simulink model "problem2"  (R2016a)
settings: Solver=VariableStepAuto  StartTime=0.0  StopTime=10.0  RelTol=1e-3
values from neighbouring files (symbols this model uses):
  x_path = planTraj(x2_i(1),x2_f(1),time)    [main.m]    (also in main_1.m = planTraj(x2_i(1),x2_f(1), 10); main_3.m = planTraj(x2_i(1),x2_f(1),10); test.m)
  y_path = planTraj(x2_i(2),x2_f(2),time)    [main.m]    (also in main_1.m = planTraj(x2_i(2),x2_f(2),10); main_3.m = planTraj(x2_i(2),x2_f(2),10); test.m)
libraries: dspinverses x1
settings Model: Creator=nathaniel  LastModifiedBy=nathaniel
settings GRTTargetCC: GeneratePreprocessorConditionals=Use local settings

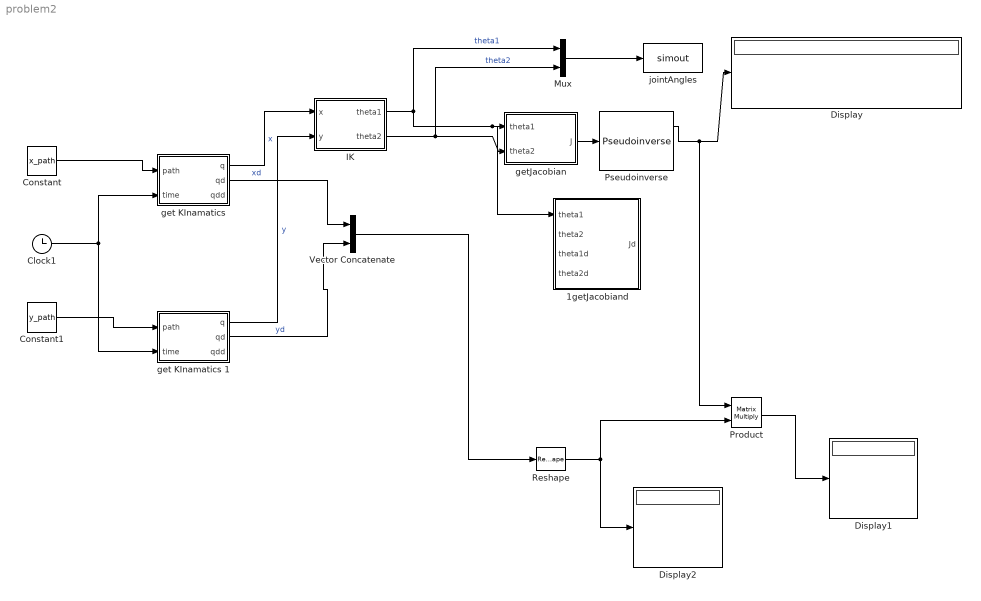
== system problem2 ==
  " 1getJacobiand " : MATLAB Function  TreatAsAtomicUnit=on
  Clock1 : Clock
  Constant : Constant  Value=x_path
  Constant1 : Constant  Value=y_path
  Display : Display
  Display1 : Display
  Display2 : Display
  "IK " : MATLAB Function  TreatAsAtomicUnit=on
  Mux : Mux  Inputs=2
  Product : Product  Multiplication=Matrix(*)
  Pseudoinverse : dspinverses/Pseudoinverse  wanterr=on
  Reshape : Reshape  OutputDimensionality=Column vector (2-D)
  Vector Concatenate : Concatenate
  "get KInamatics " : MATLAB Function  TreatAsAtomicUnit=on
  get KInamatics 1 : MATLAB Function  TreatAsAtomicUnit=on
  getJacobian : MATLAB Function  TreatAsAtomicUnit=on
  jointAngles : ToWorkspace  VariableName=simout  SaveFormat=Structure With Time  SampleTime=-1
  wires:
  Clock1/1 -> get KInamatics 1/2(time), "get KInamatics "/2(time)
  Constant1/1 -> get KInamatics 1/1(path)
  Constant/1 -> "get KInamatics "/1(path)
  get KInamatics 1/1(q) -> "IK "/2(y)  "y"
  "get KInamatics "/1(q) -> "IK "/1(x)  "x"
  "IK "/1(theta1) -> " 1getJacobiand "/1(theta1), getJacobian/1(theta1), Mux/1  "theta1"
  "IK "/2(theta2) -> getJacobian/2(theta2), Mux/2  "theta2"
  getJacobian/1(J) -> Pseudoinverse/1
  Pseudoinverse/1 -> Product/1, Display/1
  Mux/1 -> jointAngles/1
  "get KInamatics "/2(qd) -> Vector Concatenate/1  "xd"
  get KInamatics 1/2(qd) -> Vector Concatenate/2  "yd"
  Vector Concatenate/1 -> Reshape/1
  Product/1 -> Display1/1
  Reshape/1 -> Product/2, Display2/1

== matlab function problem2/get KInamatics 1 ==
  data: path input; q output; time input; qd output; qdd output
function [ q,qd,qdd] = fcn(path, time)
%#codegen
[q qd qdd] = getKin(path, time)

== matlab function problem2/get KInamatics  ==
  data: path input; q output; time input; qd output; qdd output
function [ q,qd,qdd] = fcn(path, time)
%#codegen
[q qd qdd] = getKin(path, time)

== matlab function problem2/IK  ==
  data: x input; theta1 output; y input; theta2 output
function [ theta1, theta2] = fcn(x, y)
%#codegen
[theta1 theta2] = IK(x, y)

== matlab function problem2/getJacobian ==
  data: theta1 input; J output; theta2 input
function J  = fcn(theta1, theta2)
%#codegen
J = getJacobian(theta1,theta2);

== matlab function problem2/ 1getJacobiand  ==
  data: theta1 input; theta2 input; theta1d input; Jd output; theta2d input
function Jd  = fcn(theta1,theta2, theta1d, theta2d)
%#codegen
Jd = getJacobiandot(theta1,theta1d,theta2,theta2d);
